simulink model "Modulation"  (R2021a)
settings: configuration reference "Configuration" (kept outside this file)
settings Model: DataDictionary=ZC_EVPowerSystem.sldd  Creator=ykamatan  LastModifiedBy=ykamatan
settings ConfigSetRef: SourceName=Configuration

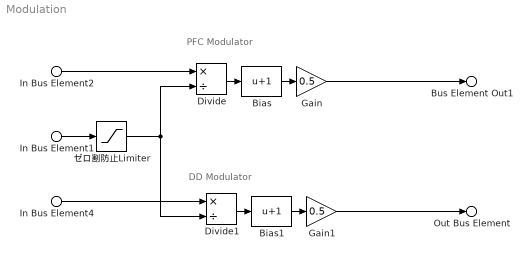
== system Modulation ==
  note: DD Modulator
  note: PFC Modulator
  In Bus Element1 : Inport  PortName=PFC_FBSig  Element=PFC_FBSig.vdc
  In Bus Element4 : Inport  Port=2  PortName=DDRef  Element=vHB
  In Bus Element2 : Inport  Port=3  PortName=PFCRef  Element=vInv
  Bias : Bias  Bias=1
  Bias1 : Bias  Bias=1
  Divide : Product  Inputs=*/
  Divide1 : Product  Inputs=*/
  Gain : Gain  Gain=0.5
  Gain1 : Gain  Gain=0.5
  ゼロ割防止Limiter : Saturate  UpperLimit=inf  LowerLimit=300
  Bus Element Out1 : Outport  PortName=PWM_Signals  Element=PFC_Duty
  Out Bus Element : Outport  PortName=PWM_Signals  Element=DD48v_Duty
  wires:
  In Bus Element4/1 -> Divide1/1
  Divide/1 -> Bias/1
  Divide1/1 -> Bias1/1
  Bias1/1 -> Gain1/1
  Gain1/1 -> Out Bus Element/1
  ゼロ割防止Limiter/1 -> Divide/2, Divide1/2
  Bias/1 -> Gain/1
  Gain/1 -> Bus Element Out1/1
  In Bus Element1/1 -> ゼロ割防止Limiter/1
  In Bus Element2/1 -> Divide/1
